simulink model "H8_2GDL_lineal"  (R2022b)
settings: Solver=VariableStepAuto  StartTime=0.0  StopTime=5  RelTol=1e-3
InitFcn:
  | load("hems.mat");
  | airgap = hems.Airgap;
  | current = hems.Current;
  | forceV = hems.Force_Vertical;
  | forceH = hems.Force_Horizontal;
  | inductance = hems.Inductance;
  | resistance = hems.Resistance;
  | 
  | m = 200;
  | g = 9.81;
  | Iyy = 26.887;
  | x_lev12 = 0.443;
  | x_lev34 = 0.542;
  | z_max = 0.0225;
  | z_min = 0.01;
  | z_nom = 0.01965;
  | I_max = 50;
  | I_min = -50;
  | 
  | suelo = 0.0225;
  | techo = 0.01;
  | lev_nom = 0.01965;
  | time_stp = 2;
values from neighbouring files (symbols this model uses):
  A2 = argout.a    [linealizacion_2gdl.m]    (also in matrices_lineal_2gdl.mat = [0 0 689.948845287 37.4788996561 0 0 139.394129714 757.14948)
  B2 = argout.b    [linealizacion_2gdl.m]    (also in matrices_lineal_2gdl.mat = [0  0; 0  0; 0.151630617985  -0.185516467151; -0.09202917439)
  C2 = argout.c    [linealizacion_2gdl.m]    (also in matrices_lineal_2gdl.mat = [1 0 0 0 0 1 0 0 0 0 1 0 ... (16 elements, 4x4)])
  D2 = argout.d    [linealizacion_2gdl.m]    (also in matrices_lineal_2gdl.mat = [0  0; 0  0; 0  0; 0  0])
  Ka = [2091.38390024  -4523.40229407  65.4441805385  -70.1021906971  152.84626499  -886.851041867; -2276.61485995  -4503.65754193  -11.1725652788  -71.2004310761  -295.543801408  -714.324235622]    [Ka.mat]    (also in linealizacion_2gdl.m = place(Aa,Ba,[-5 -4 -2+2j -2-2j -3+1j -3-1j]))
undefined symbols (not defined in the file or in its folder): hems
libraries: slpidlib x2
settings Model: Creator=USUARIO  LastModifiedBy=ramuj

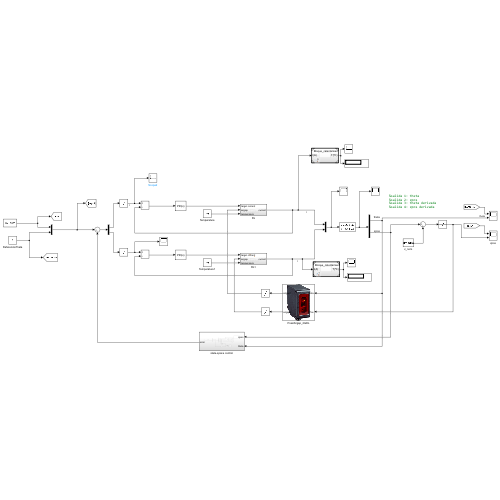
[thumbnail: Simulink's stored preview of the top-level diagram]
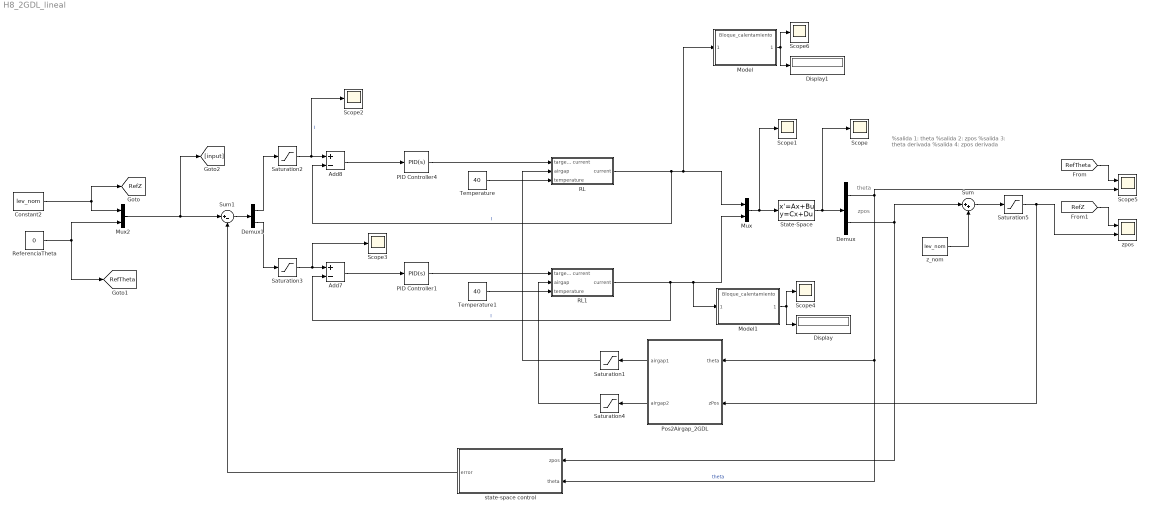
== system H8_2GDL_lineal ==
  note: zpos
  note: theta
  note: %salida 1: theta
      | %salida 2: zpos
      | %salida 3: theta derivada
      | %salida 4: zpos derivada
  Add7 : Sum  Inputs=+-
  Add8 : Sum  Inputs=+-
  Constant2 : Constant  Value=lev_nom
  Demux : Demux  Outputs=2
  Demux1 : Demux  Outputs=2
  Display : Display
  Display1 : Display
  Model : ModelReference  ModelNameDialog=Bloque_calentamiento.slx  SimulationMode=Normal  ModelReferenceVersion=3.3
  Model1 : ModelReference  ModelNameDialog=Bloque_calentamiento.slx  SimulationMode=Normal  ModelReferenceVersion=3.3
  Mux : Mux  Inputs=2
  Mux2 : Mux  Inputs=2
  PID Controller1 : slpidlib/PID Controller  Controller=PID  Form=Parallel  TimeDomain=Continuous-time  UseExternalTs=off  SampleTime=-1  IntegratorMethod=Forward Euler  FilterMethod=Forward Euler  ControllerParametersSource=internal  P=50  I=400  UseKiTs=off  D=0  N=0  UseFilter=on  TunerSelectOption=Transfer Function Based (PID Tuner App)  InitialConditionSource=internal  InitialConditionForIntegrator=0  InitialConditionForFilter=0  DifferentiatorICPrevScaledInput=0  ExternalReset=none  TrackingMode=off  Kt=1  LimitOutput=off  SatLimitsSource=internal  UpperSaturationLimit=inf  LowerSaturationLimit=-inf  LinearizeAsGain=on  AntiWindupMode=none  Kb=1  LimitIntegrator=off  UpperIntegratorSaturationLimit=inf  LowerIntegratorSaturationLimit=-inf  POutMin=[]  POutMax=[]  IOutMin=[]  IOutMax=[]  DOutMin=[]  DOutMax=[]  NOutMin=[]  NOutMax=[]  SumOutMin=[]  SumOutMax=[]  SaturationOutMin=[]  SaturationOutMax=[]  PParamMin=[]  PParamMax=[]  IParamMin=[]  IParamMax=[]  DParamMin=[]  DParamMax=[]  NParamMin=[]  NParamMax=[]  KbParamMin=[]  KbParamMax=[]  KtParamMin=[]  KtParamMax=[]  KbOutMin=[]  KbOutMax=[]  KtOutMin=[]  KtOutMax=[]  IntegratorOutMin=[]  IntegratorOutMax=[]  FilterOutMin=[]  FilterOutMax=[]  SumI1OutMin=[]  SumI1OutMax=[]  SumI2OutMin=[]  SumI2OutMax=[]  SumI3OutMin=[]  SumI3OutMax=[]  SumI4OutMin=[]  SumI4OutMax=[]  SumDOutMin=[]  SumDOutMax=[]  DifferentiatorOutMin=[]  DifferentiatorOutMax=[]  FilterDiffOutCoefMin=[]  FilterDiffOutCoefMax=[]  ReciprocalOutMin=[]  ReciprocalOutMax=[]  SumDenOutMin=[]  SumDenOutMax=[]  SumNumOutMin=[]  SumNumOutMax=[]  DivideOutMin=[]  DivideOutMax=[]  UdiffTsProdOutMin=[]  UdiffTsProdOutMax=[]  NTsProdOutMin=[]  NTsProdOutMax=[]  UintegralTsProdOutMin=[]  UintegralTsProdOutMax=[]  UngainTsProdOutMin=[]  UngainTsProdOutMax=[]  ClampingZeroOutDataTypeStr=Inherit: Inherit via back propagation  ClampingZeroOutMin=[]  ClampingZeroOutMax=[]  FilterDenConstantOutDataTypeStr=Inherit: Inherit via back propagation  FilterDenConstantOutMin=[]  FilterDenConstantOutMax=[]  PCopyOutDataTypeStr=Inherit: Inherit via back propagation  PCopyOutMin=[]  PCopyOutMax=[]  NCopyOutDataTypeStr=Inherit: Inherit via back propagation  NCopyOutMin=[]  NCopyOutMax=[]  IntegratorContinuousStateAttributes=''  IntegratorStateMustResolveToSignalObject=off  IntegratorRTWStateStorageClass=Auto  FilterContinuousStateAttributes=''  FilterStateMustResolveToSignalObject=off  FilterRTWStateStorageClass=Auto  ParallelPVariant=InternalParameters  IdealPVariant=Disabled  IVariant=InternalParameters  DVariant=InternalParameters  IntegratorVariant=Continuous  SatVariant=Disabled  AWVariant=Passthrough  PCopyVariant=Disabled  TRVariant=Disabled  FdbkBlocksVariant=Forward  IdealPFdbkVariant=Disabled  SatFdbkVariant=Disabled  DerivativeFilterVariant=ContFilter  NVariant=InternalParameters  NCopyVariant=Disabled  FilterICVariant=InternalICsFilter  IntegratorICVariant=InternalICs  ExternalResetVariant=Disabled  TRSumVariant=Passthrough  SumFdbkVariant=Disabled  SumVariant=Sum_PID  TsampFilterVariant=InternalTs  TsampNgainVariant=Passthrough  TsampIntegralVariant=Passthrough  ExternalSaturationOutDataTypeStr=Inherit: Same as second input
  PID Controller4 : slpidlib/PID Controller  Controller=PID  Form=Parallel  TimeDomain=Continuous-time  UseExternalTs=off  SampleTime=-1  IntegratorMethod=Forward Euler  FilterMethod=Forward Euler  ControllerParametersSource=internal  P=50  I=400  UseKiTs=off  D=0  N=0  UseFilter=on  TunerSelectOption=Transfer Function Based (PID Tuner App)  InitialConditionSource=internal  InitialConditionForIntegrator=0  InitialConditionForFilter=0  DifferentiatorICPrevScaledInput=0  ExternalReset=none  TrackingMode=off  Kt=1  LimitOutput=off  SatLimitsSource=internal  UpperSaturationLimit=inf  LowerSaturationLimit=-inf  LinearizeAsGain=on  AntiWindupMode=none  Kb=1  LimitIntegrator=off  UpperIntegratorSaturationLimit=inf  LowerIntegratorSaturationLimit=-inf  POutMin=[]  POutMax=[]  IOutMin=[]  IOutMax=[]  DOutMin=[]  DOutMax=[]  NOutMin=[]  NOutMax=[]  SumOutMin=[]  SumOutMax=[]  SaturationOutMin=[]  SaturationOutMax=[]  PParamMin=[]  PParamMax=[]  IParamMin=[]  IParamMax=[]  DParamMin=[]  DParamMax=[]  NParamMin=[]  NParamMax=[]  KbParamMin=[]  KbParamMax=[]  KtParamMin=[]  KtParamMax=[]  KbOutMin=[]  KbOutMax=[]  KtOutMin=[]  KtOutMax=[]  IntegratorOutMin=[]  IntegratorOutMax=[]  FilterOutMin=[]  FilterOutMax=[]  SumI1OutMin=[]  SumI1OutMax=[]  SumI2OutMin=[]  SumI2OutMax=[]  SumI3OutMin=[]  SumI3OutMax=[]  SumI4OutMin=[]  SumI4OutMax=[]  SumDOutMin=[]  SumDOutMax=[]  DifferentiatorOutMin=[]  DifferentiatorOutMax=[]  FilterDiffOutCoefMin=[]  FilterDiffOutCoefMax=[]  ReciprocalOutMin=[]  ReciprocalOutMax=[]  SumDenOutMin=[]  SumDenOutMax=[]  SumNumOutMin=[]  SumNumOutMax=[]  DivideOutMin=[]  DivideOutMax=[]  UdiffTsProdOutMin=[]  UdiffTsProdOutMax=[]  NTsProdOutMin=[]  NTsProdOutMax=[]  UintegralTsProdOutMin=[]  UintegralTsProdOutMax=[]  UngainTsProdOutMin=[]  UngainTsProdOutMax=[]  ClampingZeroOutDataTypeStr=Inherit: Inherit via back propagation  ClampingZeroOutMin=[]  ClampingZeroOutMax=[]  FilterDenConstantOutDataTypeStr=Inherit: Inherit via back propagation  FilterDenConstantOutMin=[]  FilterDenConstantOutMax=[]  PCopyOutDataTypeStr=Inherit: Inherit via back propagation  PCopyOutMin=[]  PCopyOutMax=[]  NCopyOutDataTypeStr=Inherit: Inherit via back propagation  NCopyOutMin=[]  NCopyOutMax=[]  IntegratorContinuousStateAttributes=''  IntegratorStateMustResolveToSignalObject=off  IntegratorRTWStateStorageClass=Auto  FilterContinuousStateAttributes=''  FilterStateMustResolveToSignalObject=off  FilterRTWStateStorageClass=Auto  ParallelPVariant=InternalParameters  IdealPVariant=Disabled  IVariant=InternalParameters  DVariant=InternalParameters  IntegratorVariant=Continuous  SatVariant=Disabled  AWVariant=Passthrough  PCopyVariant=Disabled  TRVariant=Disabled  FdbkBlocksVariant=Forward  IdealPFdbkVariant=Disabled  SatFdbkVariant=Disabled  DerivativeFilterVariant=ContFilter  NVariant=InternalParameters  NCopyVariant=Disabled  FilterICVariant=InternalICsFilter  IntegratorICVariant=InternalICs  ExternalResetVariant=Disabled  TRSumVariant=Passthrough  SumFdbkVariant=Disabled  SumVariant=Sum_PID  TsampFilterVariant=InternalTs  TsampNgainVariant=Passthrough  TsampIntegralVariant=Passthrough  ExternalSaturationOutDataTypeStr=Inherit: Same as second input
  Pos2Airgap_2GDL : Subsystem
      mask Display: image('C:\Users\ramuj\Desktop\Hyperloop\H8\Levitation-Repository\Levitation-Control-Dynamics\Modelo H8\image_airgapSensor.png'); % Use "Edit Image" on toolstrip to change.
  RL : Subsystem
  RL1 : Subsystem
  ReferenciaTheta : Constant  Value=0
  Saturation1 : Saturate  UpperLimit=suelo  LowerLimit=techo
  Saturation2 : Saturate  UpperLimit=I_max  LowerLimit=I_min
  Saturation3 : Saturate  UpperLimit=I_max  LowerLimit=I_min
  Saturation4 : Saturate  UpperLimit=suelo  LowerLimit=techo
  Saturation5 : Saturate  UpperLimit=suelo  LowerLimit=techo
  Scope{,1..4,6} (6 alike) : Scope
  Scope5 : Scope  NumInputPorts=2
  State-Space : StateSpace  A=A2  B=B2  C=C2  D=D2  InitialCondition=[0, suelo-lev_nom, 0, 0]
  Sum : Sum  Inputs=|++
  Sum1 : Sum  Inputs=|+-
  Temperature : Constant  Value=40
  Temperature1 : Constant  Value=40
  state-space control : Subsystem
  z_nom : Constant  Value=lev_nom
  zpos : Scope  NumInputPorts=2
  tag scope: RefTheta=global, RefZ=global
  wires:
  PID Controller1/1 -> RL1/1(target current)
  Saturation3/1 -> Scope3/1, Add7/1
  RL/1(current) -> Add8/2, Model/1, Mux/1  "I"
  PID Controller4/1 -> RL/1(target current)
  Demux/1 -> state-space control/2(theta), Pos2Airgap_2GDL/1(theta), Scope5/2  "theta"
  Saturation2/1 -> Scope2/1, Add8/1  "I"
  State-Space/1 -> Demux/1, Scope/1
  Mux/1 -> Scope1/1, State-Space/1
  RL1/1(current) -> Add7/2, Mux/2, Model1/1  "I"
  Sum/1 -> Saturation5/1
  z_nom/1 -> Sum/2
  Temperature/1 -> RL/3(temperature)
  Temperature1/1 -> RL1/3(temperature)
  Constant2/1 -> [RefZ], Mux2/1
  ReferenciaTheta/1 -> Mux2/2, [RefTheta]
  Mux2/1 -> [input], Sum1/1
  Demux1/1 -> Saturation2/1
  Demux1/2 -> Saturation3/1
  [RefTheta] -> Scope5/1
  [RefZ] -> zpos/1
  Add8/1 -> PID Controller4/1
  Add7/1 -> PID Controller1/1
  Demux/2 -> state-space control/1(zpos), Sum/1
  Pos2Airgap_2GDL/1(airgap1) -> Saturation1/1
  Pos2Airgap_2GDL/2(airgap2) -> Saturation4/1
  Sum1/1 -> Demux1/1
  Saturation1/1 -> RL/2(airgap)
  Saturation4/1 -> RL1/2(airgap)
  Saturation5/1 -> Pos2Airgap_2GDL/2(zPos), zpos/2
  state-space control/1(error) -> Sum1/2
  Model1/1 -> Scope4/1, Display/1
  Model/1 -> Scope6/1, Display1/1

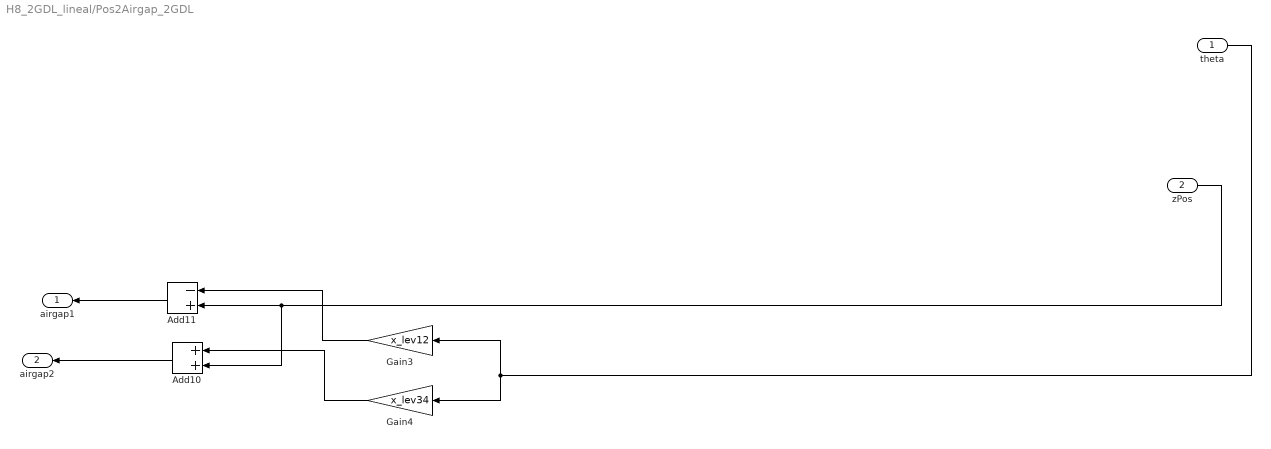
== system H8_2GDL_lineal/Pos2Airgap_2GDL ==
  theta : Inport
  zPos : Inport  Port=2
  Add10 : Sum
  Add11 : Sum  Inputs=-+
  Gain3 : Gain  Gain=x_lev12
  Gain4 : Gain  Gain=x_lev34
  airgap1 : Outport
  airgap2 : Outport  Port=2
  wires:
  Add10/1 -> airgap2/1
  zPos/1 -> Add11/2, Add10/2
  theta/1 -> Gain4/1, Gain3/1
  Gain3/1 -> Add11/1
  Gain4/1 -> Add10/1
  Add11/1 -> airgap1/1

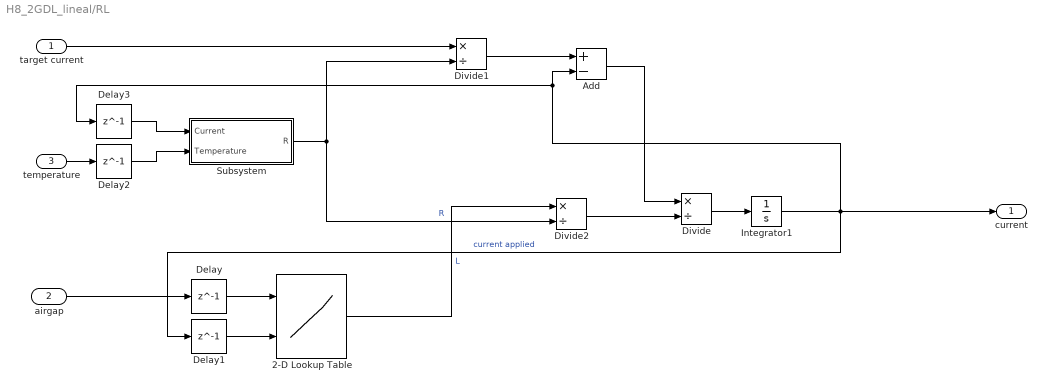
== system H8_2GDL_lineal/RL ==
  target current : Inport
  airgap : Inport  Port=2
  temperature : Inport  Port=3
  2-D Lookup Table : Lookup_n-D  BreakpointsForDimension1=hems.Airgap  BreakpointsForDimension2=hems.Current(2:110)  Table=hems.Inductance  InternalRulePriority=Speed  RndMeth=Simplest
      settings: InputPortMap=u0,u1
  Add : Sum  Inputs=+-
  Delay{,1..3} (4 alike) : Delay  DelayLength=1
  Divide : Product  Inputs=*/
  Divide1 : Product  Inputs=*/
  Divide2 : Product  Inputs=*/
  Integrator1 : Integrator
  Subsystem : Subsystem
  current : Outport
  wires:
  airgap/1 -> Delay/1
  Divide/1 -> Integrator1/1
  Add/1 -> Divide/1
  Integrator1/1 -> Delay1/1, current/1, Delay3/1, Add/2  "current applied"
  2-D Lookup Table/1 -> Divide2/1  "L"
  target current/1 -> Divide1/1
  temperature/1 -> Delay2/1
  Divide1/1 -> Add/1
  Subsystem/1(R) -> Divide2/2, Divide1/2  "R"
  Delay3/1 -> Subsystem/1(Current)
  Delay2/1 -> Subsystem/2(Temperature)
  Divide2/1 -> Divide/2
  Delay1/1 -> 2-D Lookup Table/2
  Delay/1 -> 2-D Lookup Table/1

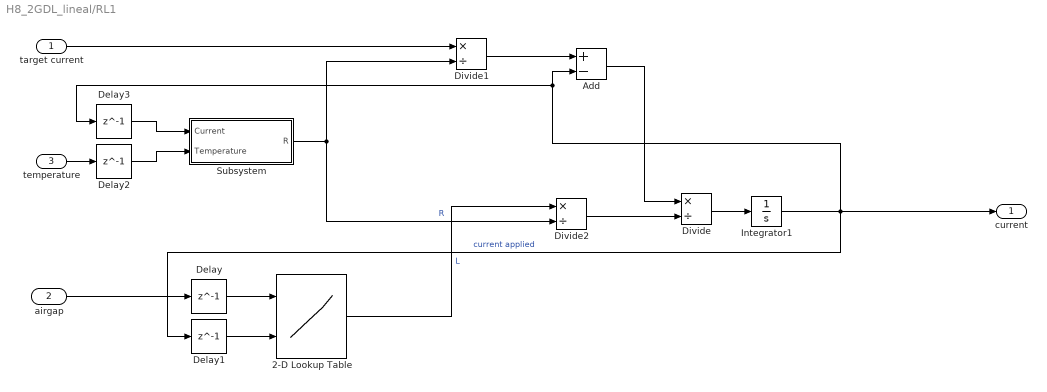
== system H8_2GDL_lineal/RL1 ==
  target current : Inport
  airgap : Inport  Port=2
  temperature : Inport  Port=3
  2-D Lookup Table : Lookup_n-D  BreakpointsForDimension1=hems.Airgap  BreakpointsForDimension2=hems.Current(2:110)  Table=hems.Inductance  InternalRulePriority=Speed  RndMeth=Simplest
      settings: InputPortMap=u0,u1
  Add : Sum  Inputs=+-
  Delay{,1..3} (4 alike) : Delay  DelayLength=1
  Divide : Product  Inputs=*/
  Divide1 : Product  Inputs=*/
  Divide2 : Product  Inputs=*/
  Integrator1 : Integrator
  Subsystem : Subsystem
  current : Outport
  wires:
  airgap/1 -> Delay/1
  Divide/1 -> Integrator1/1
  Add/1 -> Divide/1
  Integrator1/1 -> Delay1/1, current/1, Delay3/1, Add/2  "current applied"
  2-D Lookup Table/1 -> Divide2/1  "L"
  target current/1 -> Divide1/1
  temperature/1 -> Delay2/1
  Divide1/1 -> Add/1
  Subsystem/1(R) -> Divide2/2, Divide1/2  "R"
  Delay3/1 -> Subsystem/1(Current)
  Delay2/1 -> Subsystem/2(Temperature)
  Divide2/1 -> Divide/2
  Delay1/1 -> 2-D Lookup Table/2
  Delay/1 -> 2-D Lookup Table/1

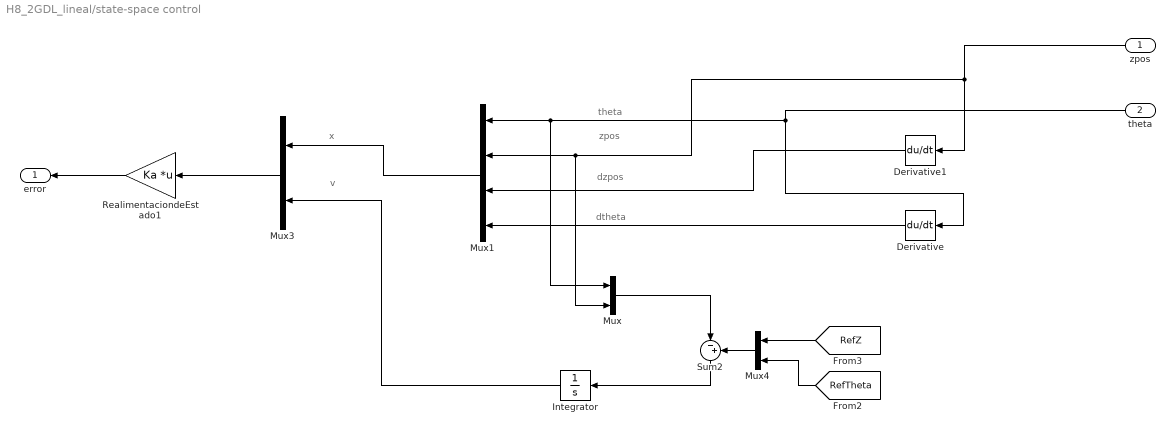
== system H8_2GDL_lineal/state-space control ==
  note: v
  note: x
  note: dtheta
  note: dzpos
  note: zpos
  note: theta
  zpos : Inport
  theta : Inport  Port=2
  Derivative : Derivative
  Derivative1 : Derivative
  Integrator : Integrator
  Mux : Mux  Inputs=2
  Mux1 : Mux
  Mux3 : Mux  Inputs=2
  Mux4 : Mux  Inputs=2
  RealimentaciondeEstado1 : Gain  Gain=Ka  Multiplication=Matrix(K*u)
  Sum2 : Sum  Inputs=|-+
  error : Outport
  wires:
  [RefZ] -> Mux4/1
  Derivative1/1 -> Mux1/3
  zpos/1 -> Mux/2, Mux1/2, Derivative1/1
  Mux4/1 -> Sum2/2
  Sum2/1 -> Integrator/1
  Mux3/1 -> RealimentaciondeEstado1/1
  theta/1 -> Derivative/1, Mux/1, Mux1/1
  [RefTheta] -> Mux4/2
  Integrator/1 -> Mux3/2
  Derivative/1 -> Mux1/4
  Mux1/1 -> Mux3/1
  RealimentaciondeEstado1/1 -> error/1
  Mux/1 -> Sum2/1

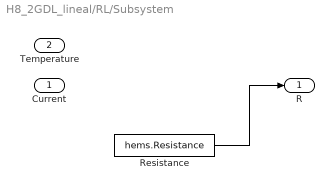
== system H8_2GDL_lineal/RL/Subsystem ==
  Current : Inport
  Temperature : Inport  Port=2
  Resistance : Constant  Value=hems.Resistance
  R : Outport
  wires:
  Resistance/1 -> R/1

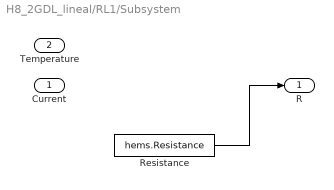
== system H8_2GDL_lineal/RL1/Subsystem ==
  Current : Inport
  Temperature : Inport  Port=2
  Resistance : Constant  Value=hems.Resistance
  R : Outport
  wires:
  Resistance/1 -> R/1
